simulink model "HW02_4"  (R2018a)
settings: Solver=VariableStepAuto  StartTime=0.0  StopTime=10.0  RelTol=1e-3
libraries: simulink x1
settings Model: Creator=lenovo  LastModifiedBy=lenovo

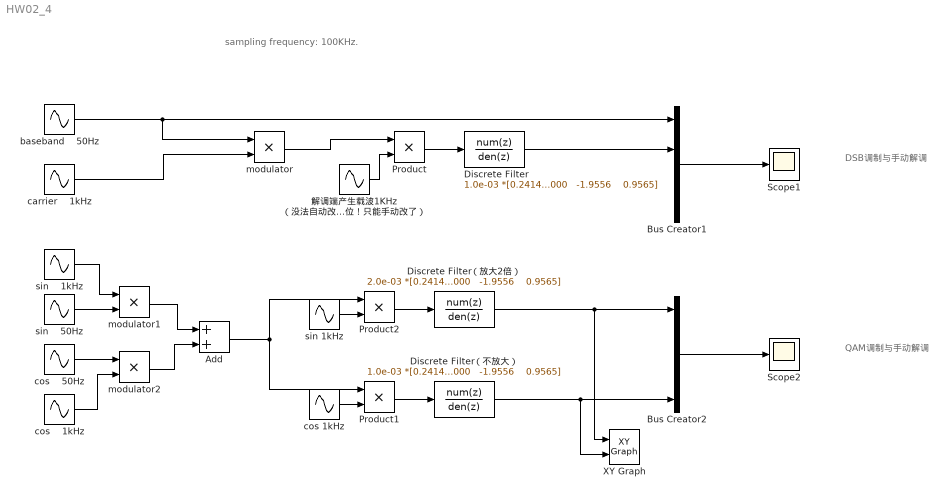
== system HW02_4 ==
  note: sampling frequency: 100KHz.
  note: DSB调制与手动解调
  note: QAM调制与手动解调
  Add : Sum
  Bus Creator1 : BusCreator  Inputs=4
  Bus Creator2 : BusCreator  Inputs=4
  Discrete Filter : DiscreteFilter  Numerator="1.0e-03 *[0.2414    0.4827    0.2414]"  Denominator="[1.0000   -1.9556    0.9565]"
  Discrete Filter（不放大） : DiscreteFilter  Numerator="1.0e-03 *[0.2414    0.4827    0.2414]"  Denominator="[1.0000   -1.9556    0.9565]"
  Discrete Filter（放大2倍） : DiscreteFilter  Numerator="2.0e-03 *[0.2414    0.4827    0.2414]"  Denominator="[1.0000   -1.9556    0.9565]"
  Product : Product
  Product1 : Product
  Product2 : Product
  Scope1 : Scope
  Scope2 : Scope
  XY Graph : simulink/Sinks/XY Graph  xmin=-1.5  xmax=1.5  ymin=-1.5  ymax=1.5  st=-1
  "baseband    50Hz  " : Sin  SineType=Sample based  Samples=2e3  SampleTime=1e-5  Offset=5e2
  "carrier    1kHz  " : Sin  SineType=Sample based  Samples=1e2  SampleTime=1e-5  Offset=25
  cos    1kHz : Sin  SineType=Sample based  Samples=1e2  SampleTime=1e-5  Offset=25
  cos    50Hz : Sin  SineType=Sample based  Samples=2e3  SampleTime=1e-5  Offset=5e2
  cos 1kHz : Sin  SineType=Sample based  Frequency=2000*pi  Samples=1e2  SampleTime=1e-5  Offset=25
  "modulator " : Product  Inputs=**
  modulator1 : Product  Inputs=**
  modulator2 : Product  Inputs=**
  sin    1kHz : Sin  SineType=Sample based  Samples=1e2  SampleTime=1e-5
  sin    50Hz : Sin  SineType=Sample based  Samples=2e3  SampleTime=1e-5
  sin 1kHz : Sin  SineType=Sample based  Frequency=2000*pi  Samples=1e2  SampleTime=1e-5
  解调端产生载波1KHz （没法自动改频率改相位！只能手动改了） : Sin  SineType=Sample based  Frequency=2000*pi  Samples=100  SampleTime=1e-5  Offset=25
  wires:
  "modulator "/1 -> Product/1
  "carrier    1kHz  "/1 -> "modulator "/2
  "baseband    50Hz  "/1 -> Bus Creator1/1, "modulator "/1
  Bus Creator1/1 -> Scope1/1
  解调端产生载波1KHz （没法自动改频率改相位！只能手动改了）/1 -> Product/2
  Product/1 -> Discrete Filter/1
  Discrete Filter/1 -> Bus Creator1/2
  Product1/1 -> Discrete Filter（不放大）/1
  Bus Creator2/1 -> Scope2/1
  cos 1kHz/1 -> Product1/2
  sin    1kHz/1 -> modulator1/1
  sin    50Hz/1 -> modulator1/2
  cos    50Hz/1 -> modulator2/1
  cos    1kHz/1 -> modulator2/2
  modulator1/1 -> Add/1
  modulator2/1 -> Add/2
  sin 1kHz/1 -> Product2/2
  Product2/1 -> Discrete Filter（放大2倍）/1
  Add/1 -> Product2/1, Product1/1
  Discrete Filter（不放大）/1 -> XY Graph/2, Bus Creator2/4
  Discrete Filter（放大2倍）/1 -> XY Graph/1, Bus Creator2/1
